simulink model "Ejer6_LimitacionFuente"  (R2023b)
settings: Solver=FixedStepDiscrete  StartTime=1  StopTime=100  FixedStep=1  RelTol=1e-3
settings Model: Creator=alfre  LastModifiedBy=alfre

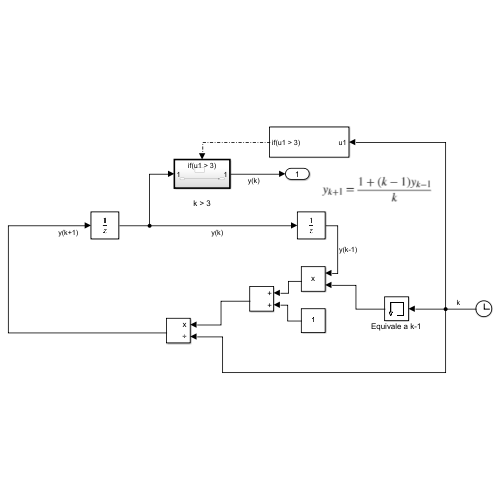
[thumbnail: Simulink's stored preview of the top-level diagram]
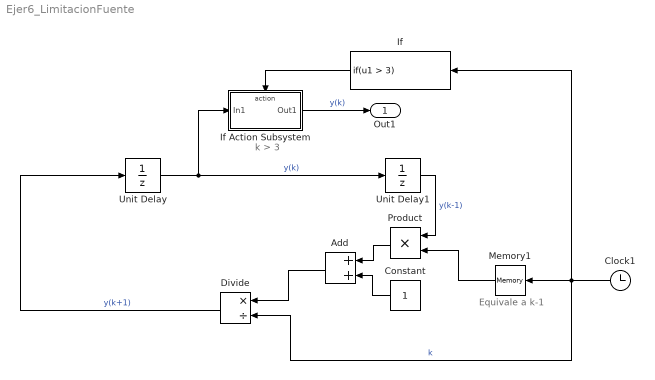
== system Ejer6_LimitacionFuente ==
  note: k > 3
  note: Equivale a k-1
  Add : Sum
  Clock1 : Clock
  Constant : Constant
  Divide : Product  Inputs=*/
  If : If  IfExpression=u1 > 3  ShowElse=off
  If Action Subsystem : Subsystem  TreatAsAtomicUnit=on
  Memory1 : Memory
  Product : Product
  Unit Delay : UnitDelay  SampleTime=-1  HasFrameUpgradeWarning=on
  Unit Delay1 : UnitDelay  SampleTime=-1  HasFrameUpgradeWarning=on
  Out1 : Outport
  wires:
  Unit Delay/1 -> Unit Delay1/1, If Action Subsystem/1(In1)  "y(k)"
  Divide/1 -> Unit Delay/1  "y(k+1)"
  Unit Delay1/1 -> Product/1  "y(k-1)"
  Constant/1 -> Add/2
  Add/1 -> Divide/1
  Product/1 -> Add/1
  Clock1/1 -> Memory1/1, Divide/2, If/1  "k"
  Memory1/1 -> Product/2
  If Action Subsystem/1(Out1) -> Out1/1  "y(k)"
  If/1 -> If Action Subsystem/Action

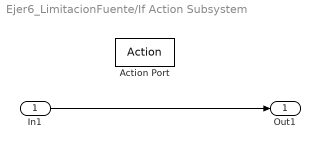
== system Ejer6_LimitacionFuente/If Action Subsystem ==
  In1 : Inport
  Action Port : ActionPort  ActionPortLabel=if(u1 > 3)
  Out1 : Outport
  wires:
  In1/1 -> Out1/1
